simulink model "robman_sim"  (Simulink 7.2)
settings: Solver=ode45  StartTime=0  StopTime=tfin  MinStep=1e-6  RelTol=1e-3
values from neighbouring files (symbols this model uses):
  robot = jacobian(robot, q)    [contactforce.m]    (also in dirkin.m = robotIn; dyn.m = dynmodel2(robot,q,dq,Ftool); dynmodel.m = neinit(robotIn,q); dynmodel2.m = neinit(robotIn,q))
undefined symbols (not defined in the file or in its folder): bDer, ctrlparam, dq0, env, q0
settings Model: Creator=Cupec  LastModifiedBy=Cupec
settings OptimizationCC: InitFltsAndDblsToZero=on
settings DebuggingCC: SaveWithParameterizedLinksMsg=none  SignalResolutionControl=TryResolveAllWithWarning  SolverPrmCheckMsg=none  MultiTaskDSMMsg=warning  MultiTaskCondExecSysMsg=none  StrictBusMsg=None
settings HardwareCC: TargetUnknown=on
settings RTWCC: IncludeERTFirstTime=on
settings GRTTargetCC: TargetFcnLib=ansi_tfl_tmw.mat

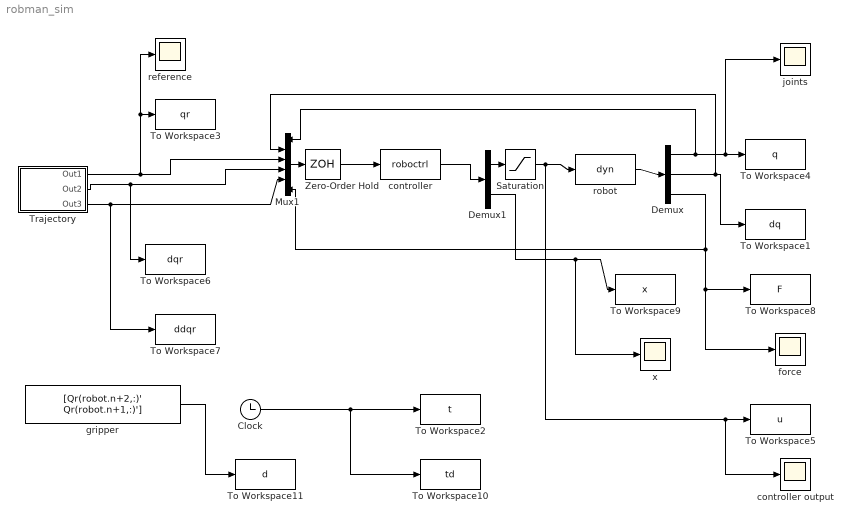
== system robman_sim ==
  Clock : Clock
  Demux : Demux  Outputs=[robot.n robot.n 6]
  Demux1 : Demux  Outputs=[robot.n ctrlparam.nStates]
  Mux1 : Mux  Inputs=6
  Saturation : Saturate  UpperLimit=ctrlparam.umax  LowerLimit=ctrlparam.umin  ZeroCross=off
  To Workspace1 : ToWorkspace  VariableName=dq  SampleTime=-1  SaveFormat=Array
  To Workspace10 : ToWorkspace  VariableName=td  SampleTime=ctrlparam.T  SaveFormat=Array
  To Workspace11 : ToWorkspace  VariableName=d  SampleTime=-1  SaveFormat=Array
  To Workspace2 : ToWorkspace  VariableName=t  SampleTime=-1  SaveFormat=Array
  To Workspace3 : ToWorkspace  VariableName=qr  SampleTime=-1  SaveFormat=Array
  To Workspace4 : ToWorkspace  VariableName=q  SampleTime=-1  SaveFormat=Array
  To Workspace5 : ToWorkspace  VariableName=u  SampleTime=-1  SaveFormat=Array
  To Workspace6 : ToWorkspace  VariableName=dqr  SampleTime=-1  SaveFormat=Array
  To Workspace7 : ToWorkspace  VariableName=ddqr  SampleTime=-1  SaveFormat=Array
  To Workspace8 : ToWorkspace  VariableName=F  SampleTime=-1  SaveFormat=Array
  To Workspace9 : ToWorkspace  VariableName=x  SampleTime=-1  SaveFormat=Array
  Trajectory : Subsystem
  Zero-Order Hold : ZeroOrderHold  SampleTime=ctrlparam.T
  controller : S-Function  FunctionName=roboctrl  Parameters=robot,ctrlparam  EnableBusSupport=off
  controller output : Scope
      settings: TimeRange=5.436  YMin=-400000  YMax=1.1e+006
  force : Scope
      settings: YMin=-19  YMax=0  SaveName=ScopeData2
  gripper : FromWorkspace  VariableName=[Qr(robot.n+2,:)' Qr(robot.n+1,:)']  SampleTime=0
  joints : Scope
      settings: TimeRange=5.436  YMin=-2.5  YMax=4
  reference : Scope
      settings: YMin=-2.5  YMax=4  SaveName=ScopeData3
  robot : S-Function  FunctionName=dyn  Parameters=robot,q0(1:robot.n),dq0,env  EnableBusSupport=off
  x : Scope
      settings: YMin=132.5  YMax=180  SaveName=ScopeData4
  wires:
  Clock/1 -> To Workspace2/1, To Workspace10/1
  robot/1 -> Demux/1
  Demux/1 -> Mux1/1, To Workspace4/1, joints/1
  Demux/2 -> To Workspace1/1, Mux1/2
  Saturation/1 -> robot/1, To Workspace5/1, controller output/1
  Trajectory/1(Out1) -> Mux1/3, To Workspace3/1, reference/1
  Trajectory/2(Out2) -> Mux1/4, To Workspace6/1
  Mux1/1 -> Zero-Order Hold/1
  Zero-Order Hold/1 -> controller/1
  Trajectory/3(Out3) -> Mux1/5, To Workspace7/1
  Demux/3 -> To Workspace8/1, force/1, Mux1/6
  Demux1/1 -> Saturation/1
  Demux1/2 -> To Workspace9/1, x/1
  gripper/1 -> To Workspace11/1
  controller/1 -> Demux1/1

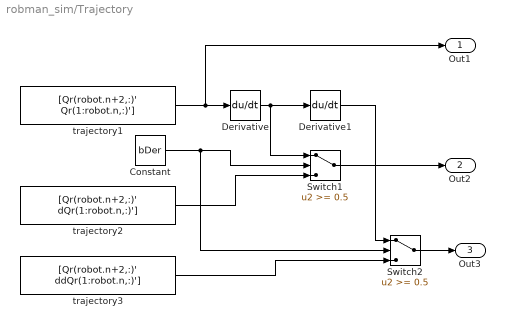
== system robman_sim/Trajectory ==
  Constant : Constant  Value=bDer  OutDataType=sfix(16)  OutScaling=2^0
  Derivative : Derivative
  Derivative1 : Derivative
  Switch1 : Switch  Threshold=0.5
  Switch2 : Switch  Threshold=0.5
  trajectory1 : FromWorkspace  VariableName=[Qr(robot.n+2,:)' Qr(1:robot.n,:)']  SampleTime=0
  trajectory2 : FromWorkspace  VariableName=[Qr(robot.n+2,:)' dQr(1:robot.n,:)']  SampleTime=0
  trajectory3 : FromWorkspace  VariableName=[Qr(robot.n+2,:)' ddQr(1:robot.n,:)']  SampleTime=0
  Out1 : Outport  OutDataType=sfix(16)  OutScaling=2^0
  Out2 : Outport  Port=2  OutDataType=sfix(16)  OutScaling=2^0
  Out3 : Outport  Port=3  OutDataType=sfix(16)  OutScaling=2^0
  wires:
  trajectory1/1 -> Derivative/1, Out1/1
  Derivative/1 -> Derivative1/1, Switch1/1
  trajectory2/1 -> Switch1/3
  Switch1/1 -> Out2/1
  Derivative1/1 -> Switch2/1
  trajectory3/1 -> Switch2/3
  Switch2/1 -> Out3/1
  Constant/1 -> Switch1/2, Switch2/2
